simulink model "quadcopter"  (R2020a)
settings: Solver=VariableStepAuto  StartTime=0.0  StopTime=10.0  RelTol=1e-3
model workspace (MAT data in the model file):
  motor_gain = 1
libraries: simulink x5
settings Model: Creator=lauri  LastModifiedBy=lauri

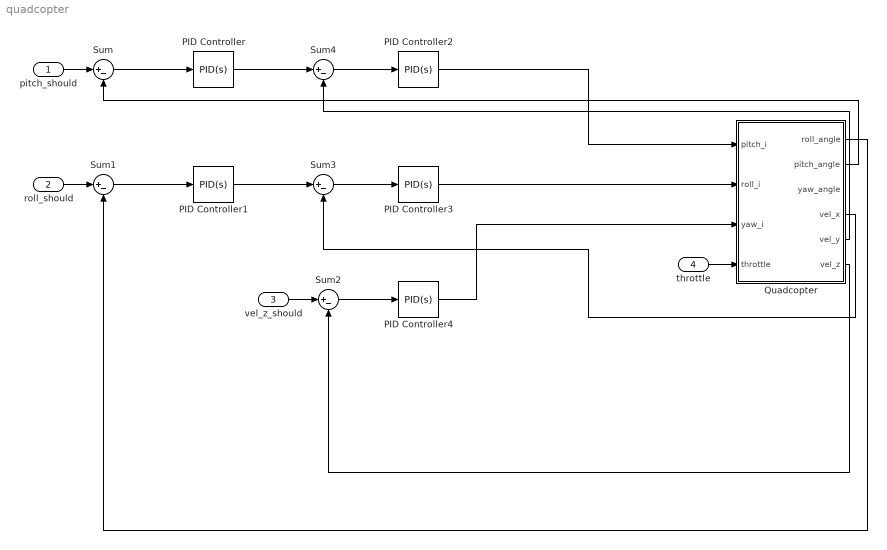
== system quadcopter ==
  pitch_should : Inport  Tag=pitch_should
  roll_should : Inport  Port=2
  vel_z_should : Inport  Port=3
  throttle : Inport  Port=4
  PID Controller{,1..4} (5 alike) : simulink/Continuous/PID Controller  Controller=PID  Form=Parallel  TimeDomain=Continuous-time  UseExternalTs=off  SampleTime=-1  IntegratorMethod=Forward Euler  FilterMethod=Forward Euler  ControllerParametersSource=internal  P=1  I=1  D=0  UseFilter=on  N=100  TunerSelectOption=Transfer Function Based (PID Tuner App)  InitialConditionSource=internal  InitialConditionForIntegrator=0  InitialConditionForFilter=0  DifferentiatorICPrevScaledInput=0  ExternalReset=none  TrackingMode=off  Kt=1  LimitOutput=off  UpperSaturationLimit=inf  LowerSaturationLimit=-inf  LinearizeAsGain=on  AntiWindupMode=none  Kb=1  POutMin=[]  POutMax=[]  IOutMin=[]  IOutMax=[]  DOutMin=[]  DOutMax=[]  NOutMin=[]  NOutMax=[]  SumOutMin=[]  SumOutMax=[]  SaturationOutMin=[]  SaturationOutMax=[]  PParamMin=[]  PParamMax=[]  IParamMin=[]  IParamMax=[]  DParamMin=[]  DParamMax=[]  NParamMin=[]  NParamMax=[]  KbParamMin=[]  KbParamMax=[]  KtParamMin=[]  KtParamMax=[]  KbOutMin=[]  KbOutMax=[]  KtOutMin=[]  KtOutMax=[]  IntegratorOutMin=[]  IntegratorOutMax=[]  FilterOutMin=[]  FilterOutMax=[]  SumI1OutMin=[]  SumI1OutMax=[]  SumI2OutMin=[]  SumI2OutMax=[]  SumI3OutMin=[]  SumI3OutMax=[]  SumI4OutMin=[]  SumI4OutMax=[]  SumDOutMin=[]  SumDOutMax=[]  DifferentiatorOutMin=[]  DifferentiatorOutMax=[]  FilterDiffOutCoefMin=[]  FilterDiffOutCoefMax=[]  ReciprocalOutMin=[]  ReciprocalOutMax=[]  SumDenOutMin=[]  SumDenOutMax=[]  SumNumOutMin=[]  SumNumOutMax=[]  DivideOutMin=[]  DivideOutMax=[]  UdiffTsProdOutMin=[]  UdiffTsProdOutMax=[]  NTsProdOutMin=[]  NTsProdOutMax=[]  UintegralTsProdOutMin=[]  UintegralTsProdOutMax=[]  UngainTsProdOutMin=[]  UngainTsProdOutMax=[]  IntegratorContinuousStateAttributes=''  IntegratorStateMustResolveToSignalObject=off  IntegratorRTWStateStorageClass=Auto  FilterContinuousStateAttributes=''  FilterStateMustResolveToSignalObject=off  FilterRTWStateStorageClass=Auto  ParallelPVariant=InternalParameters  IdealPVariant=Disabled  IVariant=InternalParameters  DVariant=InternalParameters  IntegratorVariant=Continuous  SatVariant=Disabled  AWVariant=Passthrough  PCopyVariant=Disabled  TRVariant=Disabled  FdbkBlocksVariant=Forward  IdealPFdbkVariant=Disabled  SatFdbkVariant=Disabled  DerivativeFilterVariant=ContFilter  NVariant=InternalParameters  NCopyVariant=Disabled  FilterICVariant=InternalICsFilter  IntegratorICVariant=InternalICs  ExternalResetVariant=Disabled  TRSumVariant=Passthrough  SumFdbkVariant=Disabled  SumVariant=Sum_PID  TsampFilterVariant=InternalTs  TsampNgainVariant=Passthrough  TsampIntegralVariant=Passthrough
  Quadcopter : Subsystem
  Sum{,1..4} (5 alike) : Sum  Inputs=|+-
  wires:
  Sum/1 -> PID Controller/1
  pitch_should/1 -> Sum/1
  roll_should/1 -> Sum1/1
  Sum1/1 -> PID Controller1/1
  Quadcopter/2(pitch_angle) -> Sum/2
  Quadcopter/1(roll_angle) -> Sum1/2
  vel_z_should/1 -> Sum2/1
  Sum2/1 -> PID Controller4/1
  Quadcopter/6(vel_z) -> Sum2/2
  PID Controller1/1 -> Sum3/1
  Sum3/1 -> PID Controller3/1
  PID Controller/1 -> Sum4/1
  Sum4/1 -> PID Controller2/1
  Quadcopter/4(vel_x) -> Sum3/2
  Quadcopter/5(vel_y) -> Sum4/2
  throttle/1 -> Quadcopter/4(throttle)
  PID Controller4/1 -> Quadcopter/3(yaw_i)
  PID Controller3/1 -> Quadcopter/2(roll_i)
  PID Controller2/1 -> Quadcopter/1(pitch_i)

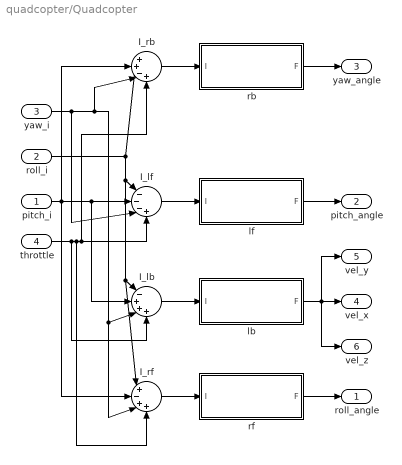
== system quadcopter/Quadcopter ==
  pitch_i : Inport
  roll_i : Inport  Port=2
  yaw_i : Inport  Port=3
  throttle : Inport  Port=4
  I_lb : Sum  Inputs=|-+++
  I_lf : Sum  Inputs=|---+
  I_rb : Sum  Inputs=|++-+
  I_rf : Sum  Inputs=|+-++
  lb : Subsystem
  lf : Subsystem
  rb : Subsystem
  rf : Subsystem
  roll_angle : Outport
  pitch_angle : Outport  Port=2
  yaw_angle : Outport  Port=3
  vel_x : Outport  Port=4
  vel_y : Outport  Port=5
  vel_z : Outport  Port=6
  wires:
  I_rb/1 -> rb/1(I)
  throttle/1 -> I_rb/4, I_lf/4, I_rf/4, I_lb/4
  rf/1(F) -> roll_angle/1
  rb/1(F) -> yaw_angle/1
  I_lf/1 -> lf/1(I)
  I_lb/1 -> lb/1(I)
  lf/1(F) -> pitch_angle/1
  lb/1(F) -> vel_y/1, vel_z/1, vel_x/1
  I_rf/1 -> rf/1(I)
  yaw_i/1 -> I_rf/3, I_lb/3, I_rb/3, I_lf/3
  pitch_i/1 -> I_lf/2, I_lb/2, I_rb/2, I_rf/2
  roll_i/1 -> I_rf/1, I_lb/1, I_lf/1, I_rb/1

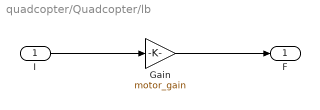
== system quadcopter/Quadcopter/lb ==
  I : Inport
  Gain : Gain  Gain=motor_gain
  F : Outport
  wires:
  I/1 -> Gain/1
  Gain/1 -> F/1

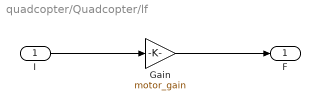
== system quadcopter/Quadcopter/lf ==
  I : Inport
  Gain : Gain  Gain=motor_gain
  F : Outport
  wires:
  I/1 -> Gain/1
  Gain/1 -> F/1

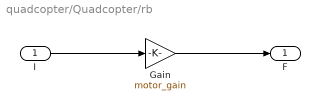
== system quadcopter/Quadcopter/rb ==
  I : Inport
  Gain : Gain  Gain=motor_gain
  F : Outport
  wires:
  I/1 -> Gain/1
  Gain/1 -> F/1

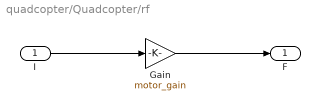
== system quadcopter/Quadcopter/rf ==
  I : Inport
  Gain : Gain  Gain=motor_gain
  F : Outport
  wires:
  I/1 -> Gain/1
  Gain/1 -> F/1
